simulink model "lqr_control"  (R2019b)
settings: Solver=FixedStepAuto  StartTime=0.0  StopTime=inf  FixedStep=0.01  RelTol=1e-3
undefined symbols (not defined in the file or in its folder): K
libraries: robotlib x8, simulink x2
settings Model: Creator=shunya  LastModifiedBy=shunya
settings OptimizationCC: EnhancedBackFolding=on  PassReuseOutputArgsAs=Individual arguments  ZeroExternalMemoryAtStartup=off  ZeroInternalMemoryAtStartup=off  MaxStackSize=64  OptimizeBlockOrder=speed  DifferentSizesBufferReuse=on  OptimizationCustomize=off  EfficientTunableParamExpr=on
settings DebuggingCC: ParameterTunabilityLossMsg=error
settings HardwareCC: ProdBitPerPointer=32  ProdBitPerSizeT=32  ProdBitPerPtrDiffT=32  ProdLargestAtomicFloat=None  ProdIntDivRoundTo=Undefined  ProdEndianess=Unspecified  ProdWordSize=32  ProdHWDeviceType=Generic->Unspecified (assume 32-bit Generic)
settings SFSimCC: MATLABDynamicMemAlloc=off
settings RTWCC: SystemTargetFile=ert.tlc  HardwareBoard=Robot Operating System (ROS)  TLCOptions="-aInlineSetEventsForThisBaseRateFcn=TLC_FALSE -aSuppressMultiTaskScheduler=TLC_FALSE  -aRateBasedStepFcn=0"  TemplateMakefile=ert_default_tmf  GenerateReport=on  Toolchain=Catkin  IncludeHyperlinkInReport=on  LaunchReport=on  TargetLang=C++  GenerateTraceInfo=on  GenerateTraceReport=on  GenerateTraceReportSl=on  GenerateTraceReportSf=on  GenerateTraceReportEml=on
settings CodeAppCC: ForceParamTrailComments=on  IgnoreCustomStorageClasses=off  OperatorAnnotations=on  SimulinkDataObjDesc=on  SFDataObjDesc=on  InsertBlockDesc=on

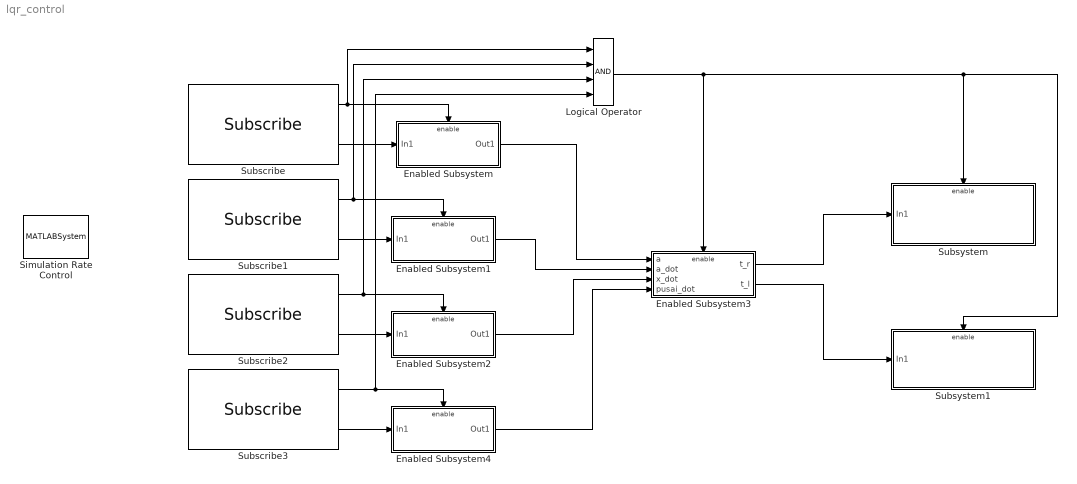
== system lqr_control ==
  Enabled Subsystem : Subsystem  TreatAsAtomicUnit=on
  Enabled Subsystem1 : Subsystem  TreatAsAtomicUnit=on
  Enabled Subsystem2 : Subsystem  TreatAsAtomicUnit=on
  Enabled Subsystem3 : Subsystem  TreatAsAtomicUnit=on
  Enabled Subsystem4 : Subsystem  TreatAsAtomicUnit=on
  Logical Operator : Logic  Inputs=4  AllPortsSameDT=off  OutDataTypeStr=boolean
  Simulation Rate Control : MATLABSystem  System=ExampleHelperSimulationRateControl  SampleTime=0.01
      mask Type: ExampleHelperSimulationRateControl
      mask Display: disp('Rate Control');
  Subscribe : robotlib/Subscribe  topicSource=Specify your own  topic=/balance_state_angle  messageType=std_msgs/Float64  sampleTime=-1  messageQueueLength=1
      settings: SourceProductName=ROS Toolbox
  Subscribe1 : robotlib/Subscribe  topicSource=Select from ROS network  topic=/balance_state_angular  messageType=std_msgs/Float64  sampleTime=-1  messageQueueLength=1
      settings: SourceProductName=ROS Toolbox
  Subscribe2 : robotlib/Subscribe  topicSource=Select from ROS network  topic=/balance_state_velocity  messageType=std_msgs/Float64  sampleTime=-1  messageQueueLength=1
      settings: SourceProductName=ROS Toolbox
  Subscribe3 : robotlib/Subscribe  topicSource=Select from ROS network  topic=/balance_state_pusai  messageType=std_msgs/Float64  sampleTime=-1  messageQueueLength=1
      settings: SourceProductName=ROS Toolbox
  Subsystem : Subsystem
  Subsystem1 : Subsystem
  wires:
  Subscribe/2 -> Enabled Subsystem/1(In1)
  Subscribe/1 -> Logical Operator/1, Enabled Subsystem/Enable
  Subscribe1/1 -> Logical Operator/2, Enabled Subsystem1/Enable
  Subscribe1/2 -> Enabled Subsystem1/1(In1)
  Subscribe2/2 -> Enabled Subsystem2/1(In1)
  Subscribe2/1 -> Logical Operator/3, Enabled Subsystem2/Enable
  Subscribe3/1 -> Enabled Subsystem4/Enable, Logical Operator/4
  Subscribe3/2 -> Enabled Subsystem4/1(In1)
  Logical Operator/1 -> Enabled Subsystem3/Enable, Subsystem/Enable, Subsystem1/Enable
  Enabled Subsystem/1(Out1) -> Enabled Subsystem3/1(a)
  Enabled Subsystem1/1(Out1) -> Enabled Subsystem3/2(a_dot)
  Enabled Subsystem2/1(Out1) -> Enabled Subsystem3/3(x_dot)
  Enabled Subsystem4/1(Out1) -> Enabled Subsystem3/4(pusai_dot)
  Enabled Subsystem3/1(t_r) -> Subsystem/1(In1)
  Enabled Subsystem3/2(t_l) -> Subsystem1/1(In1)

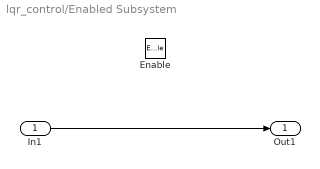
== system lqr_control/Enabled Subsystem ==
  In1 : Inport
  Enable : EnablePort
  Out1 : Outport
  wires:
  In1/1 -> Out1/1

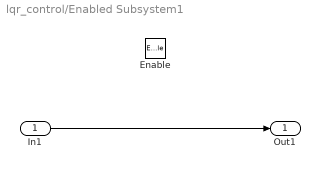
== system lqr_control/Enabled Subsystem1 ==
  In1 : Inport
  Enable : EnablePort
  Out1 : Outport
  wires:
  In1/1 -> Out1/1

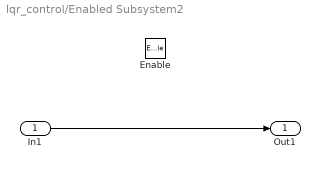
== system lqr_control/Enabled Subsystem2 ==
  In1 : Inport
  Enable : EnablePort
  Out1 : Outport
  wires:
  In1/1 -> Out1/1

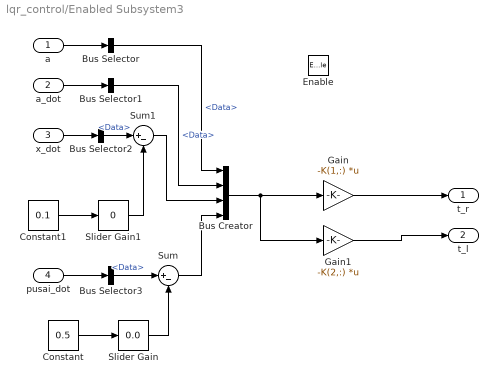
== system lqr_control/Enabled Subsystem3 ==
  a : Inport
  a_dot : Inport  Port=2
  x_dot : Inport  Port=3
  pusai_dot : Inport  Port=4
  Enable : EnablePort
  Bus Creator : BusCreator  Inputs=4
  Bus Selector{,1..3} (4 alike) : BusSelector  OutputSignals=Data
  Constant : Constant  Value=0.5
  Constant1 : Constant  Value=0.1
  Gain : Gain  Gain=-K(1,:)  Multiplication=Matrix(K*u) (u vector)
  Gain1 : Gain  Gain=-K(2,:)  Multiplication=Matrix(K*u) (u vector)
  Slider Gain : simulink/Math Operations/Slider Gain  gain=0.0  low=-1  high=1
  Slider Gain1 : simulink/Math Operations/Slider Gain  gain=0  low=-1  high=1
  Sum : Sum  Inputs=|+-
  Sum1 : Sum  Inputs=|+-
  t_r : Outport
  t_l : Outport  Port=2
  wires:
  Bus Creator/1 -> Gain1/1, Gain/1
  Gain/1 -> t_r/1
  Gain1/1 -> t_l/1
  a/1 -> Bus Selector/1
  pusai_dot/1 -> Bus Selector3/1
  x_dot/1 -> Bus Selector2/1
  a_dot/1 -> Bus Selector1/1
  Bus Selector/1 -> Bus Creator/1  "<Data>"
  Bus Selector1/1 -> Bus Creator/2  "<Data>"
  Bus Selector3/1 -> Sum/1  "<Data>"
  Constant/1 -> Slider Gain/1
  Slider Gain/1 -> Sum/2
  Sum/1 -> Bus Creator/4
  Slider Gain1/1 -> Sum1/2
  Constant1/1 -> Slider Gain1/1
  Bus Selector2/1 -> Sum1/1  "<Data>"
  Sum1/1 -> Bus Creator/3

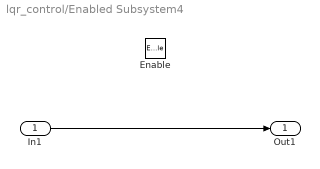
== system lqr_control/Enabled Subsystem4 ==
  In1 : Inport
  Enable : EnablePort
  Out1 : Outport
  wires:
  In1/1 -> Out1/1

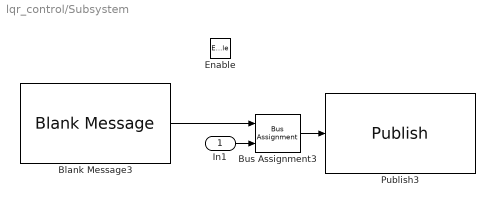
== system lqr_control/Subsystem ==
  In1 : Inport
  Enable : EnablePort
  Blank Message3 : robotlib/Blank Message  messageClass=Message  entityType=std_msgs/Float64  messageType=std_msgs/Float64  SampleTime=0.01
      settings: SourceProductName=ROS Toolbox
  Bus Assignment3 : BusAssignment  AssignedSignals=Data
  Publish3 : robotlib/Publish  topicSource=Select from ROS network  topic=/wheel_leg3/wheel1_velocity_controller/command  messageType=std_msgs/Float64  messageQueueLength=1
      settings: SourceProductName=ROS Toolbox
  wires:
  Blank Message3/1 -> Bus Assignment3/1
  Bus Assignment3/1 -> Publish3/1
  In1/1 -> Bus Assignment3/2

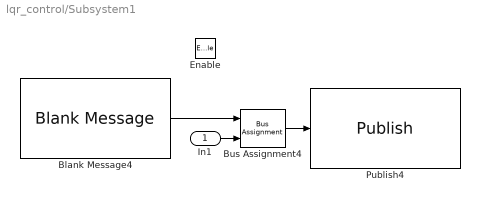
== system lqr_control/Subsystem1 ==
  In1 : Inport
  Enable : EnablePort
  Blank Message4 : robotlib/Blank Message  messageClass=Message  entityType=std_msgs/Float64  messageType=std_msgs/Float64  SampleTime=0.01
      settings: SourceProductName=ROS Toolbox
  Bus Assignment4 : BusAssignment  AssignedSignals=Data
  Publish4 : robotlib/Publish  topicSource=Select from ROS network  topic=/wheel_leg3/wheel2_velocity_controller/command  messageType=std_msgs/Float64  messageQueueLength=1
      settings: SourceProductName=ROS Toolbox
  wires:
  Bus Assignment4/1 -> Publish4/1
  In1/1 -> Bus Assignment4/2
  Blank Message4/1 -> Bus Assignment4/1
